simulink model "Mass2_sim"  (R2024a)
settings: Solver=VariableStepAuto  StartTime=0.0  StopTime=10.0  RelTol=1e-3
undefined symbols (not defined in the file): b1, b2, F, k1, k2, m1, m2
settings Model: Creator=alisr_qxy0y9  LastModifiedBy=alisr_qxy0y9

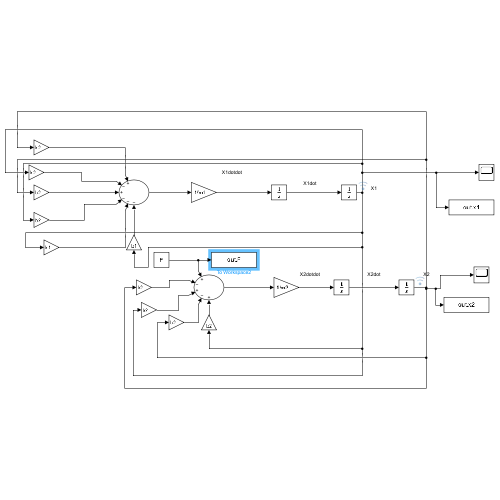
[thumbnail: Simulink's stored preview of the top-level diagram]
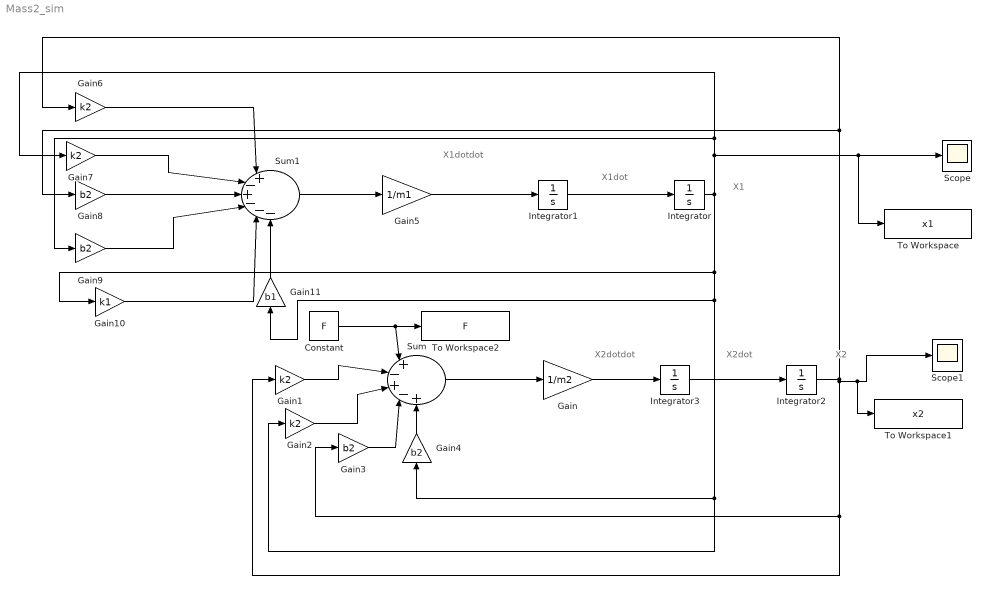
== system Mass2_sim ==
  note: X1dot
  note: X1dotdot
  note: X1
  note: X2dotdot
  note: X2dot
  note: X2
  Constant : Constant  Value=F
  Gain : Gain  Gain=1/m2
  Gain{1..2,6..7} (4 alike) : Gain  Gain=k2
  Gain10 : Gain  Gain=k1
  Gain11 : Gain  Gain=b1
  Gain{3..4,8..9} (4 alike) : Gain  Gain=b2
  Gain5 : Gain  Gain=1/m1
  Integrator{,1..3} (4 alike) : Integrator
  Scope : Scope
  Scope1 : Scope
  Sum : Sum  Inputs=|+-+-+
  Sum1 : Sum  Inputs=|+-+---
  To Workspace : ToWorkspace  VariableName=x1  SaveFormat=Timeseries  SampleTime=-1
  To Workspace1 : ToWorkspace  VariableName=x2  SaveFormat=Timeseries  SampleTime=-1
  To Workspace2 : ToWorkspace  VariableName=F  SaveFormat=Timeseries  SampleTime=-1
  wires:
  Integrator1/1 -> Integrator/1
  Integrator3/1 -> Integrator2/1
  Integrator/1 -> To Workspace/1, Scope/1, Gain9/1, Gain7/1, Gain11/1, Gain4/1, Gain2/1, Gain10/1
  Integrator2/1 -> Gain8/1, Gain6/1, Gain3/1, Gain1/1, To Workspace1/1, Scope1/1
  Sum/1 -> Gain/1
  Gain/1 -> Integrator3/1
  Constant/1 -> To Workspace2/1, Sum/1
  Gain1/1 -> Sum/2
  Gain2/1 -> Sum/3
  Gain3/1 -> Sum/4
  Gain4/1 -> Sum/5
  Gain5/1 -> Integrator1/1
  Gain6/1 -> Sum1/1
  Gain7/1 -> Sum1/2
  Gain8/1 -> Sum1/3
  Gain9/1 -> Sum1/4
  Gain10/1 -> Sum1/5
  Gain11/1 -> Sum1/6
  Sum1/1 -> Gain5/1
